simulink model "desacoplador_corrientes"  (R2023b)
settings: Solver=VariableStepAuto  StartTime=0.0  StopTime=10.0  RelTol=1e-3
values from neighbouring files (symbols this model uses):
  L_d = 6.6e-3    (= 0.0066)    [controlador_foc_simulink.m]    (also in params_subsistema_electromagnetico.m; sistema_completo_en_codigo.m)
  L_q = 5.8e-3    (= 0.0058)    [controlador_foc_simulink.m]    (also in params_subsistema_electromagnetico.m; sistema_completo_en_codigo.m)
  lambda_m = 0.016    [controlador_foc_simulink.m]    (also in parametros_planta.m; params_subsistema_electromagnetico.m; sistema_completo_en_codigo.m)
  Pp = 3    [controlador_foc_simulink.m]    (also in parametros_planta.m; params_subsistema_electromagnetico.m; sistema_completo_en_codigo.m)
settings Model: Creator=Pc  LastModifiedBy=Pc

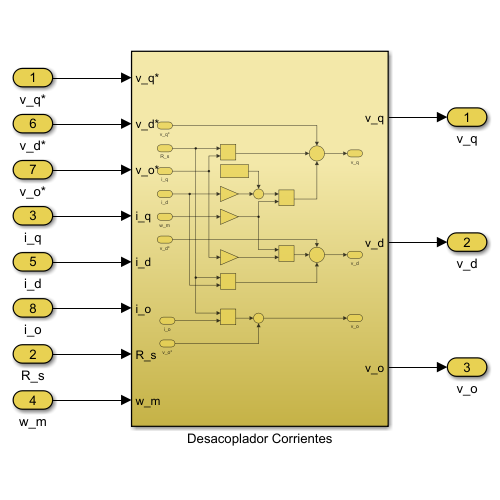
[thumbnail: Simulink's stored preview of the top-level diagram]
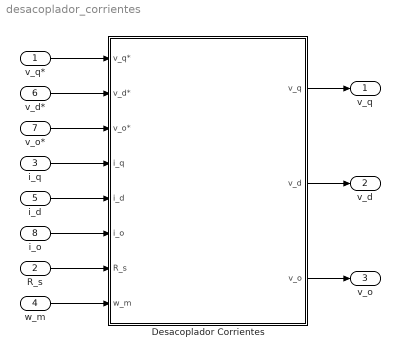
== system desacoplador_corrientes ==
  v_q* : Inport
  R_s : Inport  Port=2
  i_q : Inport  Port=3
  w_m : Inport  Port=4
  i_d : Inport  Port=5
  v_d* : Inport  Port=6
  v_o* : Inport  Port=7
  i_o : Inport  Port=8
  Desacoplador Corrientes : Subsystem
  v_q : Outport
  v_d : Outport  Port=2
  v_o : Outport  Port=3
  wires:
  v_q*/1 -> Desacoplador Corrientes/1(v_q*)
  R_s/1 -> Desacoplador Corrientes/7(R_s)
  i_q/1 -> Desacoplador Corrientes/4(i_q)
  w_m/1 -> Desacoplador Corrientes/8(w_m)
  i_d/1 -> Desacoplador Corrientes/5(i_d)
  v_d*/1 -> Desacoplador Corrientes/2(v_d*)
  v_o*/1 -> Desacoplador Corrientes/3(v_o*)
  i_o/1 -> Desacoplador Corrientes/6(i_o)
  Desacoplador Corrientes/1(v_q) -> v_q/1
  Desacoplador Corrientes/2(v_d) -> v_d/1
  Desacoplador Corrientes/3(v_o) -> v_o/1

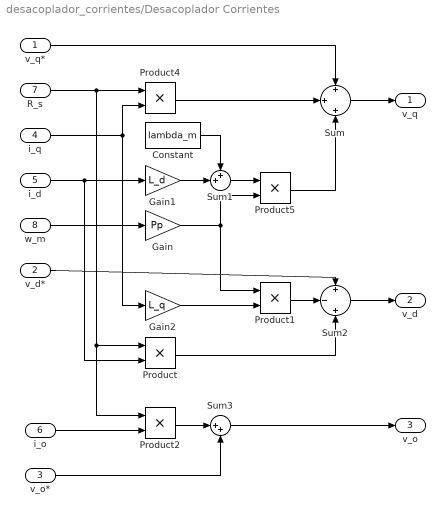
== system desacoplador_corrientes/Desacoplador Corrientes ==
  v_q* : Inport
  v_d* : Inport  Port=2
  v_o* : Inport  Port=3
  i_q : Inport  Port=4
  i_d : Inport  Port=5
  i_o : Inport  Port=6
  R_s : Inport  Port=7
  w_m : Inport  Port=8
  Constant : Constant  Value=lambda_m
  Gain : Gain  Gain=Pp
  Gain1 : Gain  Gain=L_d
  Gain2 : Gain  Gain=L_q
  Product{,1..2,4..5} (5 alike) : Product
  Sum : Sum  Inputs=+|+|+
  Sum1 : Sum  Inputs=++|
  Sum2 : Sum  Inputs=+|-|+
  Sum3 : Sum  Inputs=|++
  v_q : Outport
  v_d : Outport  Port=2
  v_o : Outport  Port=3
  wires:
  R_s/1 -> Product/1, Product2/1, Product4/1
  Product2/1 -> Sum3/1
  v_d*/1 -> Sum2/1
  Gain/1 -> Product1/1, Product5/2
  Gain1/1 -> Sum1/2
  Product/1 -> Sum2/3
  Sum3/1 -> v_o/1
  i_d/1 -> Gain1/1, Product/2
  Product5/1 -> Sum/3
  Product1/1 -> Sum2/2
  Product4/1 -> Sum/2
  v_q*/1 -> Sum/1
  i_q/1 -> Gain2/1, Product4/2
  Sum/1 -> v_q/1
  i_o/1 -> Product2/2
  Sum1/1 -> Product5/1
  Sum2/1 -> v_d/1
  v_o*/1 -> Sum3/2
  w_m/1 -> Gain/1
  Constant/1 -> Sum1/1
  Gain2/1 -> Product1/2
